simulink model "part_3"  (R2017b)
settings: Solver=VariableStepAuto  StartTime=0.0  StopTime=15  MaxStep=0.0001  MinStep=1  RelTol=1e-3
settings Model: Creator=drone  LastModifiedBy=drone
settings SolverCC: InitialStep=1

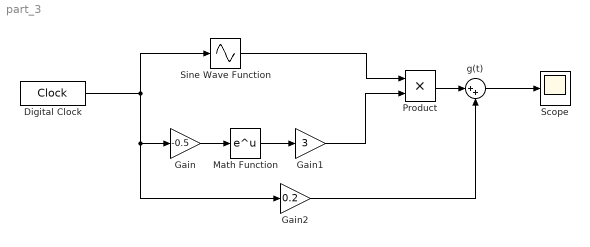
== system part_3 ==
  Digital Clock : DigitalClock  SampleTime=0.00001
  Gain : Gain  Gain=-0.5
  Gain1 : Gain  Gain=3
  Gain2 : Gain  Gain=0.2
  Math Function : Math  SaturateOnIntegerOverflow=on
  Product : Product
  Scope : Scope
  Sine Wave Function : Sin  TimeSource=Use external signal  SampleTime=0
  g(t) : Sum  Inputs=|++
  wires:
  Gain/1 -> Math Function/1
  Math Function/1 -> Gain1/1
  Sine Wave Function/1 -> Product/1
  Gain1/1 -> Product/2
  Product/1 -> g(t)/1
  Gain2/1 -> g(t)/2
  g(t)/1 -> Scope/1
  Digital Clock/1 -> Gain2/1, Gain/1, Sine Wave Function/1
